simulink model "modu"  (R2014a)
settings: Solver=ode3  StartTime=0.0  StopTime=110.0  RelTol=1e-3
undefined symbols (not defined in the file): canChannel
libraries: canlib x1
settings Model: Creator=david  LastModifiedBy=david
settings RTWCC: GenCodeOnly=on

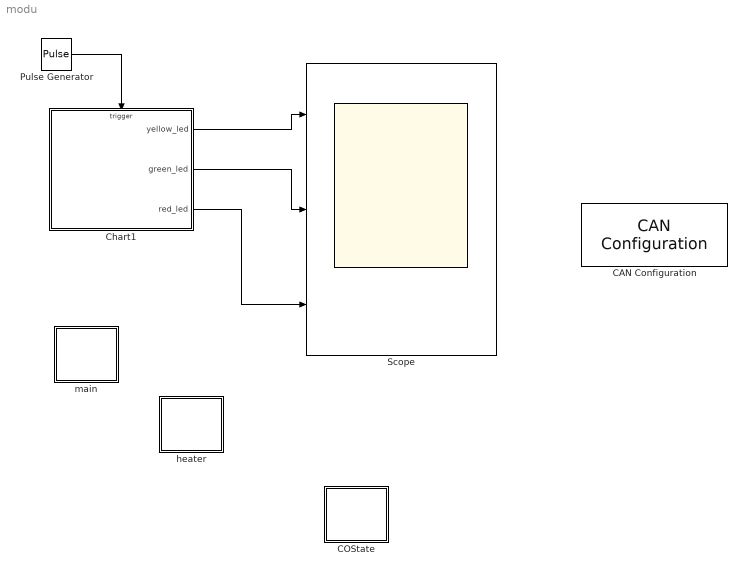
== system modu ==
  CAN Configuration : canlib/CAN Configuration  BlockHandle=3.0078  DeviceMenu=Vector Virtual 1 (Channel 1)  Device=Vector Virtual 1 (Channel 1)  ObjConstructor=canChannel('Vector', 'Virtual 1', 1)  BusSpeed=500000  EnableBitParameters=off  SJW=1  TSEG1=4  TSEG2=3  NSamples=1  AckMode=Normal
  COState : Stateflow chart  TreatAsAtomicUnit=on
  Chart1 : Stateflow chart  TreatAsAtomicUnit=on
  Pulse Generator : DiscretePulseGenerator  PulseType=Time based  Period=0.1  PulseWidth=50
  Scope : Scope  NumInputPorts=3
      settings: YMin=-5~-5~-5  YMax=5~5~5
  heater : Stateflow chart  TreatAsAtomicUnit=on
  main : Stateflow chart  TreatAsAtomicUnit=on
  wires:
  Pulse Generator/1 -> Chart1/Trigger
  Chart1/1(yellow_led) -> Scope/1
  Chart1/2(green_led) -> Scope/2
  Chart1/3(red_led) -> Scope/3

== stateflow chart modu/Chart1 ==
  state red
    entry:red_led=1;
    exit:red_led=0;
  state yellow
    entry:yellow_led=1;
    exit:yellow_led=0;
  state green
    entry:green_led=1;
    exit:green_led=0;
  (default) -> red
  yellow -> red : after(3,sec)
  red -> green : after(10,sec)
  green -> yellow : after(3,sec)
  data: yellow_led output; green_led output; red_led output
  events: tick input RISING_EDGE_EVENT

== stateflow chart modu/heater ==
  state HEATER_OFF:
    entry: give BMU control to SC
  state HEAT_BY_INV:
    entry: turn off BMU
  (default) -> HEATER_OFF:
  HEATER_OFF: -> HEAT_BY_INV: : [Tcell_min<-20]
      | and Theater<40
  HEAT_BY_INV: -> HEATER_OFF: : Tcell_min>0
      | or
      | Theart_1>60C

== stateflow chart modu/main ==
  state STANDBY:
    1) DFET/FET OFF
    2)ready to work
  state INIT:
    1) SC wakeup
    2) 2 BMU wakeup
    3) pack self check:
  state PRE_CHG:
    BMU 1 PFET on
  note: no fault
  state RUN:
    1 or 2 BMU FETs on
    state CHARGE_ONLY:
      CFET OFF,
    state NORMAL:
      DFET CFET ON
    state DCHG_ONLY:
      DFET OFF
    CHARGE_ONLY: -> NORMAL: : [OV alarm clear]
    NORMAL: -> CHARGE_ONLY: [order 1] : [UV alarm]
    NORMAL: -> DCHG_ONLY: [order 2] : [OV alarm]
    DCHG_ONLY: -> NORMAL: : [OV alarm clear]
  state FAULT
    entry: 1) all BMU DFET/CFET OFF
    2)report Fault via CAN
    3):
  state SLEEP::
    1) BMU shutdown
    2)SC shutdown
  (default) -> INIT: : [DC BUS voltage pulse?]
  (junction 24) -> PRE_CHG: [order 2] : fail, wait 3sec
  PRE_CHG: -> (junction 24)
  (junction 24) -> FAULT [order 3] : [after 3 retry ]
  (junction 24) -> NORMAL: [order 1] : success
  INIT: -> (junction 13)
  (junction 13) -> STANDBY: [order 1]
  STANDBY: -> PRE_CHG: [order 2] : get Cmd ON]
  (junction 13) -> FAULT [order 2] : [faul exist]
  FAULT -> INIT: [order 2] : [get ClrFault cmd]
  RUN: -> STANDBY: [order 1] : [get CMD_OFF]
  STANDBY: -> SLEEP:: [order 1] : 1 hour no command from TKS controller
      | or
      | lid_open/switch_off
      | or
      | E_stop command
  RUN: -> FAULT [order 3] : [any fault detected]
  RUN: -> SLEEP:: [order 2] : Lidopen
      | , Switch OFF
      | E_Stop_command
  FAULT -> SLEEP:: [order 1] : 10min
      | or
      | lidOpen detected
      | or
      | keySwitch off
      | or
      | E_Stop

== stateflow chart modu/COState ==
  state ATTACHED:
    state REQUST DETACH
    state NORMAL_OPERATION
    REQUST DETACH -> NORMAL_OPERATION : T7
    NORMAL_OPERATION -> REQUST DETACH : T6
  state DETACHED:
    state DO_NOT_ATTACH
    state READY_TO_ATTACH
    state ERROR
    ERROR -> DO_NOT_ATTACH : T10
    DO_NOT_ATTACH -> ERROR [order 2] : T11
    DO_NOT_ATTACH -> READY_TO_ATTACH [order 1] : T2
    READY_TO_ATTACH -> DO_NOT_ATTACH [order 1] : T8
    READY_TO_ATTACH -> ERROR [order 2] : T5
  (default) -> DO_NOT_ATTACH : T1
  ATTACHED: -> DO_NOT_ATTACH [order 1] : T3
  READY_TO_ATTACH -> NORMAL_OPERATION [order 3] : T4
  ATTACHED: -> ERROR [order 2] : T9
